simulink model "Pendulum_Robot_with_Motor"  (R2015a)
settings: Solver=ode15s  StartTime=0.0  StopTime=10  MaxStep=Ts  RelTol=1e-3
values from neighbouring files (symbols this model uses):
  b_phi = 0    [Setup_Parameters.m]
  b_x = 0    [Setup_Parameters.m]
  Counts_per_Revolution = 3200    [Setup_Parameters.m]
  K_gyro = (S_gyro / 1000) * (180 / pi)    (= 1.90794945779)    [Setup_Parameters.m]
  Ke = (Max_voltage - Ra*Max_RPM_Current)/(Max_RPM*2*pi/60)    (= 0.538580327423)    [Setup_Parameters.m]
  Kt = tau_max/stall_current    (= 0.240092647516)    [Setup_Parameters.m]
  Ktheta = 2*pi/Counts_per_Revolution    (= 0.00196349540849)    [Setup_Parameters.m]
  Kv = Max_voltage/Value_for_full_PWM    (= 0.0470588235294)    [Setup_Parameters.m]
  l = .38    (= 0.38)    [Setup_Parameters.m]
  La = 0    [Setup_Parameters.m]
  m1 = .6    (= 0.6)    [Setup_Parameters.m]
  m2 = 1.9    [Setup_Parameters.m]
  Max_voltage = 12    [Setup_Parameters.m]
  phi_0 = pi    (= 3.14159265359)    [Compare_full_and_linearized_models.m]    (also in Compare_full_and_linearized_models_torqueinput.m; Control_Design.m = 0; Setup_Parameters.m)
  r = Wheel_radius/39.37    (= 0.0762001524003)    [Setup_Parameters.m]
  Ra = Max_voltage/stall_current    (= 2.4)    [Setup_Parameters.m]
  Ts = .001    (= 0.001)    [Setup_Parameters.m]
  V_gyro_0 = 1.23    [Setup_Parameters.m]
  V_gyro_max = 3    [Setup_Parameters.m]
  V_gyro_min = 0    [Setup_Parameters.m]
settings Model: Creator=tvincent  LastModifiedBy=tvincent

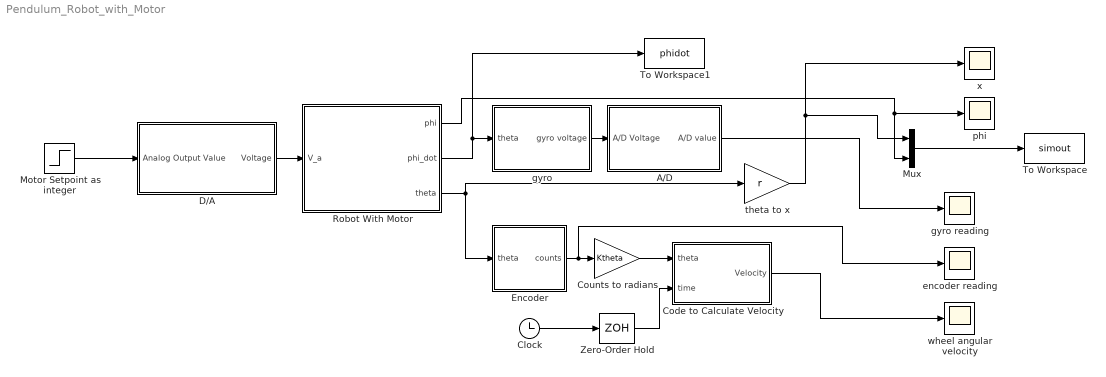
== system Pendulum_Robot_with_Motor ==
  A/D : Subsystem
  Clock : Clock
  Code to Calculate Velocity : MATLAB Function  TreatAsAtomicUnit=on
  Counts to radians : Gain  Gain=Ktheta
  D/A : Subsystem
  Encoder : Subsystem
  Motor Setpoint as integer : Step  Time=0  After=10  SampleTime=0
  Mux : Mux  Inputs=2
  Robot With Motor : Subsystem
  To Workspace : ToWorkspace  VariableName=simout  SaveFormat=Timeseries  SampleTime=Ts
  To Workspace1 : ToWorkspace  VariableName=phidot  SaveFormat=Timeseries  SampleTime=Ts
  Zero-Order Hold : ZeroOrderHold  SampleTime=Ts
  encoder reading : Scope
      settings: SaveName=ScopeData5
  gyro : Subsystem
  gyro reading : Scope
  phi : Scope
      settings: SaveName=ScopeData3
  theta to x : Gain  Gain=r
  wheel angular velocity : Scope
      settings: SaveName=ScopeData2
  x : Scope
  wires:
  Robot With Motor/2(phi_dot) -> To Workspace1/1, gyro/1(theta)
  Robot With Motor/3(theta) -> theta to x/1, Encoder/1(theta)
  Robot With Motor/1(phi) -> Mux/2, phi/1
  Mux/1 -> To Workspace/1
  Motor Setpoint as integer/1 -> D/A/1(Analog Output Value)
  D/A/1(Voltage) -> Robot With Motor/1(V_a)
  Encoder/1(counts) -> encoder reading/1, Counts to radians/1
  Clock/1 -> Zero-Order Hold/1
  Zero-Order Hold/1 -> Code to Calculate Velocity/2(time)
  Counts to radians/1 -> Code to Calculate Velocity/1(theta)
  theta to x/1 -> Mux/1, x/1
  Code to Calculate Velocity/1(Velocity) -> wheel angular velocity/1
  gyro/1(gyro voltage) -> A/D/1(A/D Voltage)
  A/D/1(A/D value) -> gyro reading/1

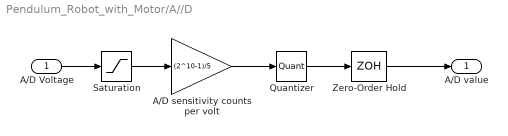
== system Pendulum_Robot_with_Motor/A//D ==
  A/D Voltage : Inport
  A/D sensitivity counts per volt : Gain  Gain=(2^10-1)/5
  Quantizer : Quantizer  QuantizationInterval=1
  Saturation : Saturate  UpperLimit=5  LowerLimit=0
  Zero-Order Hold : ZeroOrderHold  SampleTime=Ts
  A/D value : Outport
  wires:
  A/D Voltage/1 -> Saturation/1
  Zero-Order Hold/1 -> A/D value/1
  Saturation/1 -> A/D sensitivity counts per volt/1
  A/D sensitivity counts per volt/1 -> Quantizer/1
  Quantizer/1 -> Zero-Order Hold/1

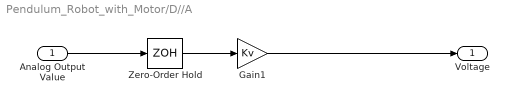
== system Pendulum_Robot_with_Motor/D//A ==
  Analog Output Value : Inport
  Gain1 : Gain  Gain=Kv
  Zero-Order Hold : ZeroOrderHold  SampleTime=Ts
  Voltage : Outport
  wires:
  Analog Output Value/1 -> Zero-Order Hold/1
  Zero-Order Hold/1 -> Gain1/1
  Gain1/1 -> Voltage/1

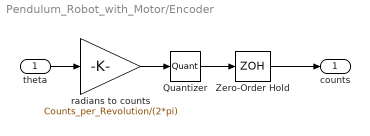
== system Pendulum_Robot_with_Motor/Encoder ==
  theta : Inport
  Quantizer : Quantizer  QuantizationInterval=1
  Zero-Order Hold : ZeroOrderHold  SampleTime=Ts
  radians to counts : Gain  Gain=Counts_per_Revolution/(2*pi)
  counts : Outport
  wires:
  Quantizer/1 -> Zero-Order Hold/1
  theta/1 -> radians to counts/1
  Zero-Order Hold/1 -> counts/1
  radians to counts/1 -> Quantizer/1

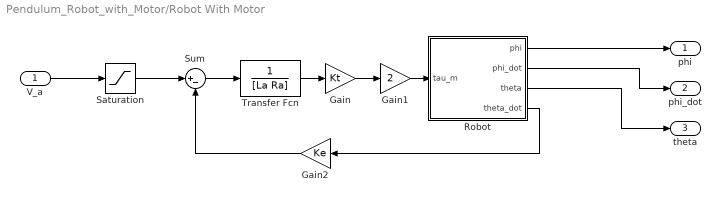
== system Pendulum_Robot_with_Motor/Robot With Motor ==
  V_a : Inport
  Gain : Gain  Gain=Kt
  Gain1 : Gain  Gain=2
  Gain2 : Gain  Gain=Ke
  Robot : Subsystem
  Saturation : Saturate  UpperLimit=Max_voltage  LowerLimit=-Max_voltage
  Sum : Sum  Inputs=|+-
  Transfer Fcn : TransferFcn  Denominator=[La Ra]
  phi : Outport
  phi_dot : Outport  Port=2
  theta : Outport  Port=3
  wires:
  Robot/2(phi_dot) -> phi_dot/1
  Gain2/1 -> Sum/2
  Robot/3(theta) -> theta/1
  Sum/1 -> Transfer Fcn/1
  Transfer Fcn/1 -> Gain/1
  Robot/1(phi) -> phi/1
  Saturation/1 -> Sum/1
  V_a/1 -> Saturation/1
  Gain/1 -> Gain1/1
  Gain1/1 -> Robot/1(tau_m)
  Robot/4(theta_dot) -> Gain2/1

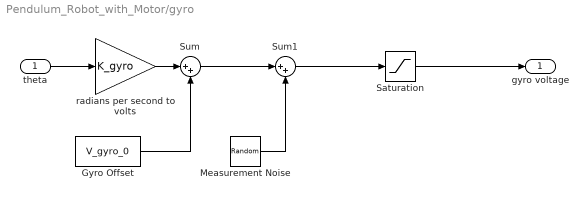
== system Pendulum_Robot_with_Motor/gyro ==
  theta : Inport
  Gyro Offset : Constant  Value=V_gyro_0
  Measurement Noise : RandomNumber  Variance=0  SampleTime=Ts
  Saturation : Saturate  UpperLimit=V_gyro_max  LowerLimit=V_gyro_min
  Sum : Sum  Inputs=|++
  Sum1 : Sum  Inputs=|++
  radians per second to volts : Gain  Gain=K_gyro
  gyro voltage : Outport
  wires:
  theta/1 -> radians per second to volts/1
  Saturation/1 -> gyro voltage/1
  radians per second to volts/1 -> Sum/1
  Gyro Offset/1 -> Sum/2
  Measurement Noise/1 -> Sum1/2
  Sum/1 -> Sum1/1
  Sum1/1 -> Saturation/1

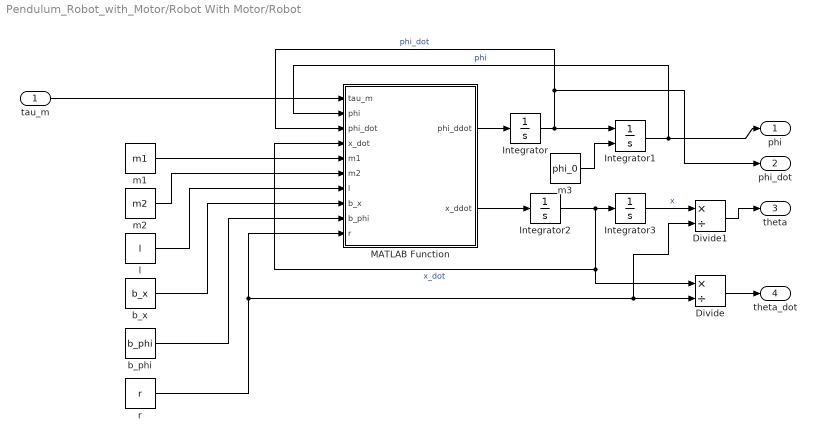
== system Pendulum_Robot_with_Motor/Robot With Motor/Robot ==
  tau_m : Inport
  Divide : Product  Inputs=*/
  Divide1 : Product  Inputs=*/
  Integrator : Integrator
  Integrator1 : Integrator  InitialConditionSource=external  InitialCondition=pi
  Integrator2 : Integrator
  Integrator3 : Integrator
  MATLAB Function : MATLAB Function  TreatAsAtomicUnit=on
  b_phi : Constant  Value=b_phi
  b_x : Constant  Value=b_x
  l : Constant  Value=l
  m1 : Constant  Value=m1
  m2 : Constant  Value=m2
  m3 : Constant  Value=phi_0
  r : Constant  Value=r
  phi : Outport
  phi_dot : Outport  Port=2
  theta : Outport  Port=3
  theta_dot : Outport  Port=4
  wires:
  Integrator2/1 -> MATLAB Function/4(x_dot), Divide/1, Integrator3/1  "x_dot"
  m1/1 -> MATLAB Function/5(m1)
  Integrator1/1 -> phi/1, MATLAB Function/2(phi)  "phi"
  MATLAB Function/1(phi_ddot) -> Integrator/1
  MATLAB Function/2(x_ddot) -> Integrator2/1
  l/1 -> MATLAB Function/7(l)
  b_x/1 -> MATLAB Function/8(b_x)
  m2/1 -> MATLAB Function/6(m2)
  b_phi/1 -> MATLAB Function/9(b_phi)
  tau_m/1 -> MATLAB Function/1(tau_m)
  r/1 -> Divide1/2, Divide/2, MATLAB Function/10(r)
  Integrator/1 -> Integrator1/1, phi_dot/1, MATLAB Function/3(phi_dot)  "phi_dot"
  Divide/1 -> theta_dot/1
  Integrator3/1 -> Divide1/1  "x"
  Divide1/1 -> theta/1
  m3/1 -> Integrator1/2

== matlab function Pendulum_Robot_with_Motor/Code to Calculate Velocity ==
  data: theta input; Velocity output; time input
function Velocity = fcn(theta,time)
%#codegen

persistent t_past;
persistent theta_past;
persistent Velocity_filt;
if isempty(t_past), t_past=0; end;
if isempty(theta_past), theta_past=0; end;
if isempty(Velocity_filt), Velocity_filt=0; end;

Ts=time-t_past;
t_past = time;
if Ts>0,
 V_d = (theta - theta_past)/Ts;
else
 V_d = 0;
end;
theta_past=theta;

Velocity_filt = .9*Velocity_filt + .1*V_d;

Velocity=Velocity_filt;

== matlab function Pendulum_Robot_with_Motor/Robot With Motor/Robot/MATLAB Function ==
  data: tau_m input; phi_ddot output; phi input; phi_dot input; x_dot input; m1 input; m2 input; l input; b_x input; b_phi input; r input; x_ddot output
function [phi_ddot,x_ddot] = phi_ddot(tau_m,phi,phi_dot,x_dot,m1,m2,l,b_x,b_phi,r)
%#codegen

g=9.81;

phi_ddot = ((g*(m1+m2) - m1*l*cos(phi)*(phi_dot)^2)*sin(phi) - cos(phi)*b_x*x_dot - ...
    ((m1+m2)/(m1*l))*b_phi*phi_dot + ((m1+m2)/(m1*l) + cos(phi)/r)*tau_m) / ...
    (l*(m2+m1*sin(phi)^2));

x_ddot = (g*m1*cos(phi)*sin(phi) - m1*l*sin(phi)*phi_dot^2 - b_x*x_dot - ...
    (cos(phi)/l)*b_phi*phi_dot + ((cos(phi)/l)+(1/r))*tau_m) / ...
    (m2+m1*sin(phi)^2);
